simulink model "tire_estimator_base"  (R2024b)
settings: Solver=VariableStepAuto  StartTime=0.0  StopTime=10.0  FixedStep=0.004  RelTol=1e-3
libraries: simulink_extras x5
settings Model: Creator=lukec  LastModifiedBy=lukec
settings SolverCC: ZeroCrossControl=DisableAll
settings OptimizationCC: DefaultParameterBehavior=Inlined  EnhancedBackFolding=on  PassReuseOutputArgsAs=Individual arguments  ZeroExternalMemoryAtStartup=off  ZeroInternalMemoryAtStartup=off  OptimizeBlockOrder=speed  DifferentSizesBufferReuse=on  OptimizationCustomize=off  EfficientTunableParamExpr=on
settings DebuggingCC: ParameterTunabilityLossMsg=error
settings HardwareCC: ProdBitPerPointer=32  ProdBitPerSizeT=32  ProdBitPerPtrDiffT=32  ProdLargestAtomicInteger=Long  ProdLargestAtomicFloat=Double  ProdWordSize=32  ProdHWDeviceType=ARM Compatible->ARM Cortex-M
settings SFSimCC: MATLABDynamicMemAlloc=off
settings RTWCC: Description=Embedded Coder  SystemTargetFile=ert.tlc  GenCodeOnly=on  PackageGeneratedCodeAndArtifacts=on  TemplateMakefile=ert_default_tmf  Toolchain=CMake  TargetLang=C++  HalideCodeGeneration=on
settings CodeAppCC: ForceParamTrailComments=on  IgnoreCustomStorageClasses=off  MaxIdLength=255  OperatorAnnotations=on  SimulinkDataObjDesc=on  SFDataObjDesc=on  InsertBlockDesc=on
settings ERTTargetCC: TargetLangStandard=C++17 (ISO)  CodeInterfacePackaging=C++ class  RootIOFormat=Structure reference  ERTCustomFileTemplate=example_file_process.tlc  ArrayContainerType=std::array

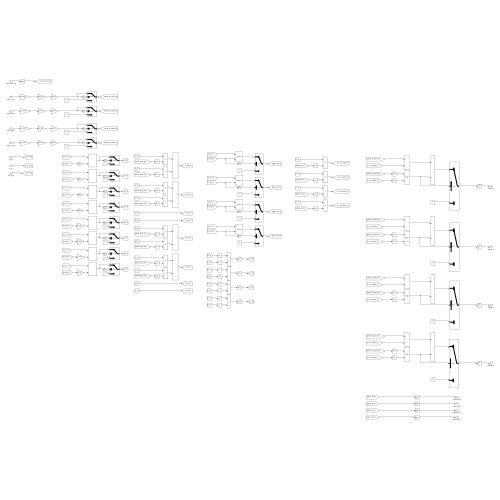
[thumbnail: Simulink's stored preview of the top-level diagram]
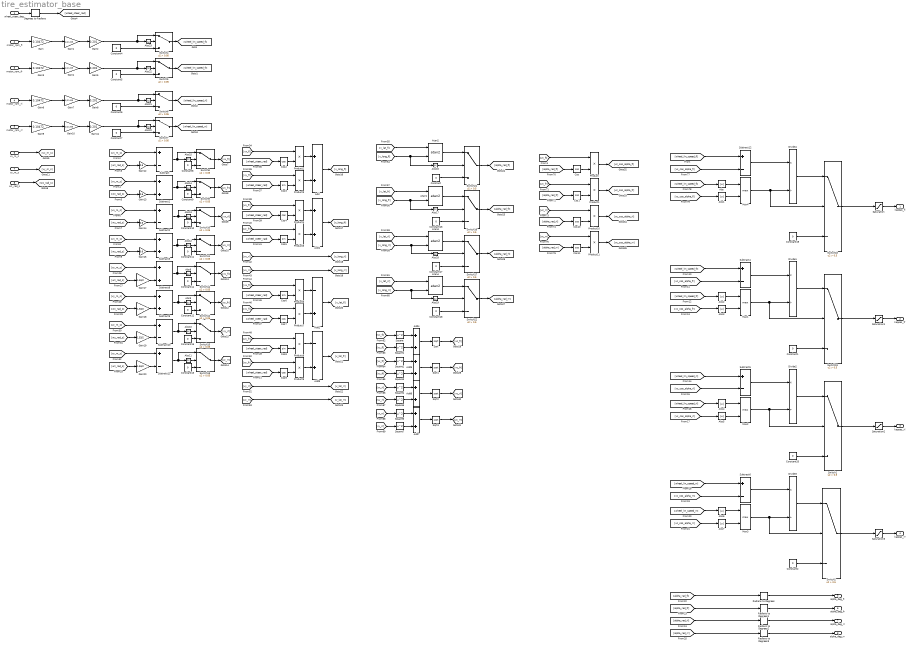
== system tire_estimator_base ==
  wheel_steer_deg : Inport
  motor_rpm_fl : Inport  Port=2
  motor_rpm_fr : Inport  Port=3
  motor_rpm_rl : Inport  Port=4
  motor_rpm_rr : Inport  Port=5
  vx_m_s : Inport  Port=6
  vy_m_s : Inport  Port=7
  wz_rad_s : Inport  Port=8
  Abs{,1..23} (24 alike) : Abs  SaturateOnIntegerOverflow=off
  Add{,1,4..7} (6 alike) : Sum
  Add2 : Sum  Inputs=-+
  Add3 : Sum  Inputs=-+
  Atan{1..4} (4 alike) : Trigonometry  Operator=atan2
  Constant{,1..2,4..20} (20 alike) : Constant  Value=0
  Cos{,1..2,4,7,9..11} (8 alike) : Trigonometry  Operator=cos
  Cos{3,5..6,8} (4 alike) : Trigonometry
  Degrees to Radians : simulink_extras/Transformations/Degrees to Radians
  Divide{1..4} (4 alike) : Product  Inputs=*/
  Gain{,3,6,9} (4 alike) : Gain  Gain=0.10472
  Gain{1,4,7,10} (4 alike) : Gain  Gain=1/11.83
  Gain{2,5,8,11} (4 alike) : Gain  Gain=0.201
  Gain{12..15} (4 alike) : Gain  Gain=0.6
  Gain{17..20} (4 alike) : Gain  Gain=1.53/2
  Max{1..4} (4 alike) : MinMax  Function=max  Inputs=2
  Product{,1..11} (12 alike) : Product
  Radians to Degrees{,1..3} (4 alike) : simulink_extras/Transformations/Radians to Degrees
  Saturation{,1..3} (4 alike) : Saturate  UpperLimit=1  LowerLimit=-1
  Sqrt{,1..3} (4 alike) : Sqrt
  Square{,1..7} (8 alike) : Math  Operator=square
  Subtract{,2,4..6,10..12} (8 alike) : Sum  Inputs=+-
  Subtract{1,3,8..9} (4 alike) : Sum
  Switch{1..2,16..19,21..22} (8 alike) : Switch  Criteria=u2 > Threshold  Threshold=0.5  SaturateOnIntegerOverflow=off  InputSameDT=off
  Switch{4..15} (12 alike) : Switch  Criteria=u2 > Threshold  Threshold=0.05  SaturateOnIntegerOverflow=off  InputSameDT=off
  kappas_fl : Outport
  kappas_fr : Outport  Port=2
  kappas_rl : Outport  Port=3
  kappas_rr : Outport  Port=4
  alpha_deg_fl : Outport  Port=5
  alpha_deg_fr : Outport  Port=6
  alpha_deg_rl : Outport  Port=7
  alpha_deg_rr : Outport  Port=8
  wires:
  motor_rpm_fl/1 -> Gain/1
  Gain/1 -> Gain1/1
  Gain1/1 -> Gain2/1
  Gain3/1 -> Gain4/1
  motor_rpm_fr/1 -> Gain3/1
  motor_rpm_rl/1 -> Gain6/1
  Gain6/1 -> Gain7/1
  Gain9/1 -> Gain10/1
  motor_rpm_rr/1 -> Gain9/1
  wheel_steer_deg/1 -> Degrees to Radians/1
  Degrees to Radians/1 -> [wheel_steer_rad]
  [vx_m_s] -> Subtract/1
  [wz_rad_s] -> Gain12/1
  Gain12/1 -> Subtract/2
  Gain13/1 -> Subtract1/2
  [wz_rad_s] -> Gain13/1
  [vx_m_s] -> Subtract1/1
  [vx_m_s] -> Subtract3/1
  [wz_rad_s] -> Gain15/1
  Gain15/1 -> Subtract3/2
  Gain14/1 -> Subtract2/2
  [wz_rad_s] -> Gain14/1
  [vx_m_s] -> Subtract2/1
  Saturation/1 -> kappas_fl/1
  Switch4/1 -> [wheel_lin_speed_fl]
  Gain2/1 -> Abs23/1, Switch4/1
  Constant4/1 -> Switch4/3
  Constant5/1 -> Switch5/3
  Gain4/1 -> Gain5/1
  Switch5/1 -> [wheel_lin_speed_fr]
  Switch6/1 -> [wheel_lin_speed_rl]
  Gain7/1 -> Gain8/1
  Constant6/1 -> Switch6/3
  Constant7/1 -> Switch7/3
  Gain10/1 -> Gain11/1
  Switch7/1 -> [wheel_lin_speed_rr]
  Subtract/1 -> Abs15/1, Switch8/1
  Constant8/1 -> Switch8/3
  Switch8/1 -> [vx_fl]
  Switch9/1 -> [vx_fr]
  Constant9/1 -> Switch9/3
  Subtract1/1 -> Abs14/1, Switch9/1
  Subtract2/1 -> Abs13/1, Switch10/1
  Constant10/1 -> Switch10/3
  Switch10/1 -> [vx_rl]
  Switch11/1 -> [vx_rr]
  Constant11/1 -> Switch11/3
  Subtract3/1 -> Abs12/1, Switch11/1
  wz_rad_s/1 -> [wz_rad_s]
  vy_m_s/1 -> [vy_m_s]
  Switch14/1 -> [vy_fl]
  Constant14/1 -> Switch14/3
  Subtract8/1 -> Abs8/1, Switch14/1
  Gain17/1 -> Subtract8/2
  [wz_rad_s] -> Gain17/1
  [vy_m_s] -> Subtract8/1
  [vy_m_s] -> Subtract9/1
  [wz_rad_s] -> Gain18/1
  Gain18/1 -> Subtract9/2
  Subtract9/1 -> Abs9/1, Switch12/1
  Constant12/1 -> Switch12/3
  Switch12/1 -> [vy_fr]
  Switch13/1 -> [vy_rr]
  Constant13/1 -> Switch13/3
  Subtract11/1 -> Abs11/1, Switch13/1
  Gain20/1 -> Subtract11/2
  [wz_rad_s] -> Gain20/1
  [vy_m_s] -> Subtract11/1
  [vy_m_s] -> Subtract10/1
  [wz_rad_s] -> Gain19/1
  Gain19/1 -> Subtract10/2
  Subtract10/1 -> Abs10/1, Switch15/1
  Constant15/1 -> Switch15/3
  Switch15/1 -> [vy_rl]
  [vx_fl] -> Product2/1
  [wheel_steer_rad] -> Cos2/1
  Cos2/1 -> Product2/2
  Cos3/1 -> Product3/2
  [wheel_steer_rad] -> Cos3/1
  [vy_fl] -> Product3/1
  Product3/1 -> Add/2
  Product2/1 -> Add/1
  Add/1 -> [v_long_fl]
  Add1/1 -> [v_long_fr]
  Product4/1 -> Add1/1
  Product5/1 -> Add1/2
  [vy_fr] -> Product5/1
  [wheel_steer_rad] -> Cos5/1
  Cos5/1 -> Product5/2
  Cos4/1 -> Product4/2
  [wheel_steer_rad] -> Cos4/1
  [vx_fr] -> Product4/1
  [vx_rl] -> [v_long_rl]
  [vx_rr] -> [v_long_rr]
  Add2/1 -> [v_lat_fl]
  Product6/1 -> Add2/1
  Product7/1 -> Add2/2
  [vy_fl] -> Product7/1
  [wheel_steer_rad] -> Cos7/1
  Cos7/1 -> Product7/2
  Cos6/1 -> Product6/2
  [wheel_steer_rad] -> Cos6/1
  [vx_fl] -> Product6/1
  [vx_fr] -> Product8/1
  [wheel_steer_rad] -> Cos8/1
  Cos8/1 -> Product8/2
  Cos9/1 -> Product9/2
  [wheel_steer_rad] -> Cos9/1
  [vy_fr] -> Product9/1
  Product9/1 -> Add3/2
  Product8/1 -> Add3/1
  Add3/1 -> [v_lat_fr]
  [vy_rr] -> [v_lat_rr]
  [vy_rl] -> [v_lat_rl]
  [v_lat_fl] -> Atan2/1
  [v_long_fl] -> Abs16/1, Atan2/2
  [v_long_fr] -> Abs17/1, Atan1/2
  [v_lat_fr] -> Atan1/1
  [v_lat_rl] -> Atan3/1
  [v_long_rl] -> Abs18/1, Atan3/2
  [v_long_rr] -> Abs19/1, Atan4/2
  [v_lat_rr] -> Atan4/1
  [vx_fl] -> Square/1
  [vy_fl] -> Square1/1
  Square/1 -> Add4/1
  Square1/1 -> Add4/2
  Add4/1 -> Sqrt/1
  Sqrt/1 -> [vc_fl]
  Sqrt1/1 -> [vc_fr]
  Add5/1 -> Sqrt1/1
  Square3/1 -> Add5/2
  Square2/1 -> Add5/1
  [vy_fr] -> Square3/1
  [vx_fr] -> Square2/1
  [vx_rl] -> Square4/1
  [vy_rl] -> Square5/1
  Square4/1 -> Add6/1
  Square5/1 -> Add6/2
  Add6/1 -> Sqrt2/1
  Sqrt2/1 -> [vc_rl]
  Sqrt3/1 -> [vc_rr]
  Add7/1 -> Sqrt3/1
  Square7/1 -> Add7/2
  Square6/1 -> Add7/1
  [vy_rr] -> Square7/1
  [vx_rr] -> Square6/1
  [wheel_lin_speed_fl] -> Subtract12/1
  [alpha_rad_fl] -> Cos/1
  Cos/1 -> Product/2
  [vc_fl] -> Product/1
  Product/1 -> [vc_cos_alpha_fl]
  Product1/1 -> [vc_cos_alpha_fr]
  [vc_fr] -> Product1/1
  Cos1/1 -> Product1/2
  [alpha_rad_fr] -> Cos1/1
  [alpha_rad_rl] -> Cos10/1
  Cos10/1 -> Product10/2
  [vc_rl] -> Product10/1
  Product10/1 -> [vc_cos_alpha_rl]
  Product11/1 -> [vc_cos_alpha_rr]
  [vc_rr] -> Product11/1
  Cos11/1 -> Product11/2
  [alpha_rad_rr] -> Cos11/1
  [vc_cos_alpha_fl] -> Subtract12/2
  Subtract12/1 -> Divide4/1
  [wheel_lin_speed_fl] -> Abs/1
  [vc_cos_alpha_fl] -> Abs1/1
  Abs/1 -> Max4/1
  Abs1/1 -> Max4/2
  Max4/1 -> Divide4/2, Switch18/2
  Max1/1 -> Switch19/2, Divide1/2
  Abs3/1 -> Max1/2
  Abs2/1 -> Max1/1
  [vc_cos_alpha_fr] -> Abs3/1
  [wheel_lin_speed_fr] -> Abs2/1
  Subtract4/1 -> Divide1/1
  [vc_cos_alpha_fr] -> Subtract4/2
  [wheel_lin_speed_fr] -> Subtract4/1
  Saturation1/1 -> kappas_fr/1
  Saturation2/1 -> kappas_rl/1
  [wheel_lin_speed_rl] -> Subtract5/1
  [vc_cos_alpha_rl] -> Subtract5/2
  Subtract5/1 -> Divide2/1
  [wheel_lin_speed_rl] -> Abs4/1
  [vc_cos_alpha_rl] -> Abs5/1
  Abs4/1 -> Max2/1
  Abs5/1 -> Max2/2
  Max2/1 -> Switch1/2, Divide2/2
  Max3/1 -> Switch2/2, Divide3/2
  Abs7/1 -> Max3/2
  Abs6/1 -> Max3/1
  [vc_cos_alpha_rr] -> Abs7/1
  [wheel_lin_speed_rr] -> Abs6/1
  Subtract6/1 -> Divide3/1
  [vc_cos_alpha_rr] -> Subtract6/2
  [wheel_lin_speed_rr] -> Subtract6/1
  Saturation3/1 -> kappas_rr/1
  [alpha_rad_fl] -> Radians to Degrees/1
  Radians to Degrees/1 -> alpha_deg_fl/1
  Radians to Degrees1/1 -> alpha_deg_fr/1
  [alpha_rad_fr] -> Radians to Degrees1/1
  [alpha_rad_rl] -> Radians to Degrees2/1
  Radians to Degrees2/1 -> alpha_deg_rl/1
  Radians to Degrees3/1 -> alpha_deg_rr/1
  [alpha_rad_rr] -> Radians to Degrees3/1
  Abs8/1 -> Switch14/2
  Abs9/1 -> Switch12/2
  Abs10/1 -> Switch15/2
  Abs11/1 -> Switch13/2
  Gain5/1 -> Abs22/1, Switch5/1
  Gain8/1 -> Abs21/1, Switch6/1
  Gain11/1 -> Abs20/1, Switch7/1
  vx_m_s/1 -> [vx_m_s]
  Abs12/1 -> Switch11/2
  Abs13/1 -> Switch10/2
  Abs14/1 -> Switch9/2
  Abs15/1 -> Switch8/2
  Abs16/1 -> Switch21/2
  Abs17/1 -> Switch16/2
  Abs18/1 -> Switch17/2
  Abs19/1 -> Switch22/2
  Abs20/1 -> Switch7/2
  Abs21/1 -> Switch6/2
  Abs22/1 -> Switch5/2
  Abs23/1 -> Switch4/2
  Switch21/1 -> [alpha_rad_fl]
  Atan2/1 -> Switch21/1
  Constant/1 -> Switch21/3
  Switch16/1 -> [alpha_rad_fr]
  Switch17/1 -> [alpha_rad_rl]
  Switch22/1 -> [alpha_rad_rr]
  Atan1/1 -> Switch16/1
  Constant16/1 -> Switch16/3
  Atan3/1 -> Switch17/1
  Constant17/1 -> Switch17/3
  Atan4/1 -> Switch22/1
  Constant18/1 -> Switch22/3
  Divide4/1 -> Switch18/1
  Switch18/1 -> Saturation/1
  Constant19/1 -> Switch18/3
  Divide1/1 -> Switch19/1
  Constant1/1 -> Switch19/3
  Switch19/1 -> Saturation1/1
  Divide2/1 -> Switch1/1
  Switch1/1 -> Saturation2/1
  Constant20/1 -> Switch1/3
  Divide3/1 -> Switch2/1
  Switch2/1 -> Saturation3/1
  Constant2/1 -> Switch2/3
